simulink model "Electromech_sys_deformation"  (R2025b)
settings: Solver=VariableStepAuto  StartTime=0.0  StopTime=10.0  RelTol=1e-3
values from neighbouring files (symbols this model uses):
  p_0 = 0    [Init_Simulink_param_nl_Electromech.m]
  phat_0 = 1e-3    (= 0.001)    [Init_Simulink_param_nl_Electromech.m]
  q_0 = 0    [Init_Simulink_param_nl_Electromech.m]
  Q_0 = 0    [Init_Simulink_param_nl_Electromech.m]
  qhat_0 = 2e-4    (= 0.0002)    [Init_Simulink_param_nl_Electromech.m]
  Qhat_0 = 5e-8    (= 5e-08)    [Init_Simulink_param_nl_Electromech.m]
undefined symbols (not defined in the file or in its folder): params
settings Model: Creator=filippougolini  LastModifiedBy=filippougolini

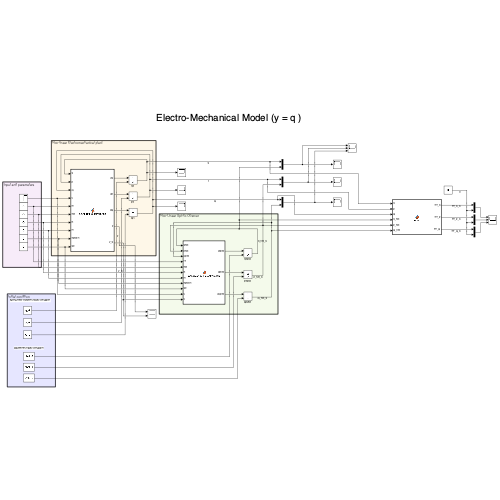
[thumbnail: Simulink's stored preview of the top-level diagram]
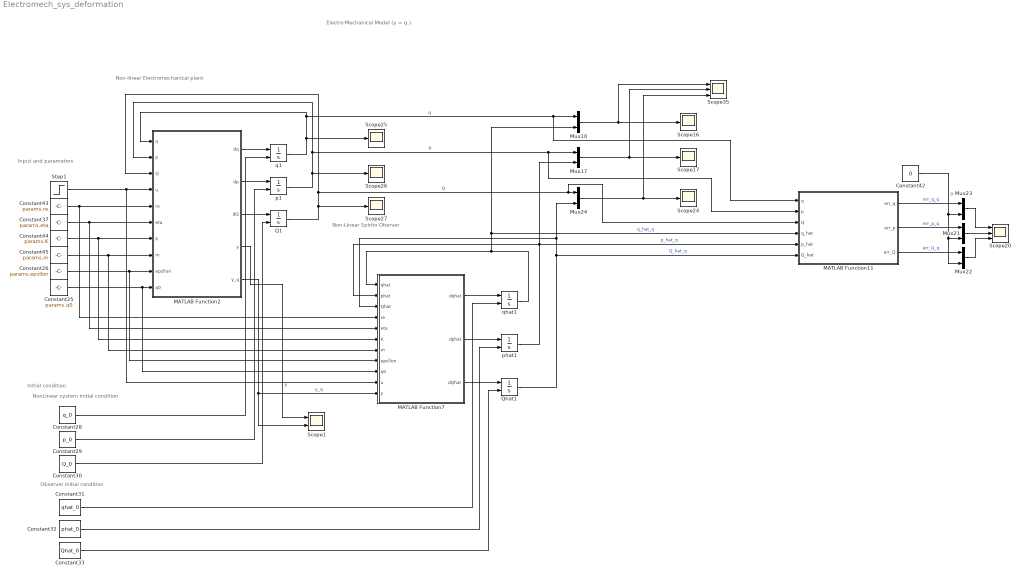
== system Electromech_sys_deformation ==
  note: Observer initial condition
  note: NonLinear system initial condition
  note: Electro-Mechanical Model (y = q )
  note: Input and parameters
  note: Non-linear Electromechanical plant
  note: Non-Linear Spirito Oberver
  note: Initial condition
  Constant25 : Constant  Value=params.q0
  Constant26 : Constant  Value=params.epsllon
  Constant28 : Constant  Value=q_0
  Constant29 : Constant  Value=p_0
  Constant30 : Constant  Value=Q_0
  Constant31 : Constant  Value=qhat_0
  Constant32 : Constant  Value=phat_0
  Constant33 : Constant  Value=Qhat_0
  Constant37 : Constant  Value=params.eta
  Constant42 : Constant  Value=0
  Constant43 : Constant  Value=params.re
  Constant44 : Constant  Value=params.K
  Constant45 : Constant  Value=params.m
  MATLAB Function11 : MATLAB Function  TreatAsAtomicUnit=on
  MATLAB Function2 : MATLAB Function  TreatAsAtomicUnit=on
  MATLAB Function7 : MATLAB Function  TreatAsAtomicUnit=on
  Mux{10,17,21..24} (6 alike) : Mux  Inputs=2
  Q1 : Integrator  InitialConditionSource=external
  Qhat1 : Integrator  InitialConditionSource=external  InitialCondition=30e-9
  Scope1 : Scope  NumInputPorts=2
      settings: ActiveDisplayYMinimum=-1  ActiveDisplayYMaximum=1
  Scope{16..17,24..27} (6 alike) : Scope
      Scope16 settings: ActiveDisplayYMinimum=-4.4929456410290065E-5  ActiveDisplayYMaximum=0.00036894675529116814  DataLoggingVariableName=ScopeData16
      Scope17 settings: ActiveDisplayYMinimum=-1  ActiveDisplayYMaximum=1  DataLoggingVariableName=ScopeData17
      Scope24 settings: ActiveDisplayYMinimum=-1  ActiveDisplayYMaximum=1  DataLoggingVariableName=ScopeData24
      Scope25 settings: ActiveDisplayYMinimum=-4.0944874698701246E-5  ActiveDisplayYMaximum=0.0003685038722883113  DataLoggingVariableName=ScopeData25
      Scope26 settings: ActiveDisplayYMinimum=-1  ActiveDisplayYMaximum=1  DataLoggingVariableName=ScopeData26
      Scope27 settings: ActiveDisplayYMinimum=-1  ActiveDisplayYMaximum=1  DataLoggingVariableName=ScopeData27
  Scope20 : Scope  NumInputPorts=3
      settings: ActiveDisplayYMinimum=-9.103686486906033E-11  ActiveDisplayYMaximum=9.2639247372251711E-11  DataLoggingVariableName=ScopeData20
  Scope35 : Scope  NumInputPorts=3
      settings: ActiveDisplayYMinimum=-4.4755980863160714E-5  ActiveDisplayYMaximum=0.00036913374297087179  DataLoggingVariableName=ScopeData35
  Step1 : Step  After=5e3  SampleTime=0
  p1 : Integrator  InitialConditionSource=external
  phat1 : Integrator  InitialConditionSource=external  InitialCondition=5e-4
  q1 : Integrator  InitialConditionSource=external
  qhat1 : Integrator  InitialConditionSource=external  InitialCondition=20e-5
  wires:
  Constant44/1 -> MATLAB Function2/7(K), MATLAB Function7/6(K)
  Constant33/1 -> Qhat1/2
  Mux17/1 -> Scope35/2, Scope17/1
  Step1/1 -> MATLAB Function7/10(u), MATLAB Function2/4(u)
  Constant37/1 -> MATLAB Function2/6(eta), MATLAB Function7/5(eta)
  MATLAB Function2/1(dq) -> q1/1
  Mux10/1 -> Scope35/1, Scope16/1
  MATLAB Function11/2(err_p) -> Mux21/1  "err_p_q"
  Constant25/1 -> MATLAB Function7/9(q0), MATLAB Function2/10(q0)
  phat1/1 -> MATLAB Function7/2(phat), MATLAB Function11/5(p_hat), Mux17/2  "p_hat_q"
  q1/1 -> Scope25/1, MATLAB Function2/1(q), Mux10/1, MATLAB Function11/1(q)  "q"
  MATLAB Function7/2(dphat) -> phat1/1
  Constant31/1 -> qhat1/2
  Constant29/1 -> p1/2
  MATLAB Function11/1(err_q) -> Mux23/1  "err_q_q"
  MATLAB Function7/1(dqhat) -> qhat1/1
  Constant45/1 -> MATLAB Function2/8(m), MATLAB Function7/7(m)
  MATLAB Function11/3(err_Q) -> Mux22/1  "err_Q_q"
  MATLAB Function7/3(dQhat) -> Qhat1/1
  Mux23/1 -> Scope20/1
  Constant32/1 -> phat1/2
  Mux21/1 -> Scope20/2
  Q1/1 -> Mux24/1, MATLAB Function11/3(Q), MATLAB Function2/3(Q), Scope27/1  "Q"
  MATLAB Function2/2(dp) -> p1/1
  Mux22/1 -> Scope20/3
  Constant30/1 -> Q1/2
  qhat1/1 -> MATLAB Function7/1(qhat), Mux10/2, MATLAB Function11/4(q_hat)  "q_hat_q"
  Constant28/1 -> q1/2
  Constant26/1 -> MATLAB Function2/9(epsllon), MATLAB Function7/8(epsllon)
  Constant43/1 -> MATLAB Function2/5(re), MATLAB Function7/4(re)
  Constant42/1 -> Mux22/2, Mux21/2, Mux23/2  "0"
  Mux24/1 -> Scope35/3, Scope24/1
  Qhat1/1 -> MATLAB Function11/6(Q_hat), Mux24/2, MATLAB Function7/3(Qhat)  "Q_hat_q"
  MATLAB Function2/3(dQ) -> Q1/1
  p1/1 -> Scope26/1, Mux17/1, MATLAB Function11/2(p), MATLAB Function2/2(p)  "p"
  MATLAB Function2/4(y) -> Scope1/1  "y"
  MATLAB Function2/5(y_q) -> Scope1/2, MATLAB Function7/11(y)  "y_q"

== matlab function Electromech_sys_deformation/MATLAB Function11 ==
  data: q input; err_q output; p input; Q input; q_hat input; p_hat input; Q_hat input; err_p output; err_Q output
function [err_q, err_p, err_Q] = error(q, p, Q, q_hat, p_hat, Q_hat)

    err_q = q - q_hat;
    err_p = p - p_hat;
    err_Q = Q - Q_hat;
end

== matlab function Electromech_sys_deformation/MATLAB Function2 ==
  data: q input; p input; Q input; u input; dq output; re input; eta input; K input; m input; epsllon input; q0 input; dp output; dQ output; y output; y_q output
function [dq, dp, dQ, y, y_q] = plant_pH_electromech(q, p, Q, u, re, eta, K, m, epsllon, q0)
% Electro-mechanical pH plant

    % Parameters: m, K, eta, eps, re, q0 in workspace

    J = [  0  1  0;
          -1  0  0;
           0  0  0 ];

    R = diag([0, eta, 1/re]);
    g = [0; 0; 1/re];

    % Hamiltonian gradient gradH(q,p,Q)
    Cq   = epsllon * (q + q0)^4;

    dHdq = K*q - 2*Q^2 / (epsllon * (q + q0)^5);
    dHdp = p / m;
    dHdQ = Q / Cq;

    gradH = [dHdq; dHdp; dHdQ];

    xdot = (J - R) * gradH + g*u;
    psi = [1/K ; 0; 2*Q/(K * (q + q0))];

    y_q = psi' * gradH; % output is the deformation
    y = q;
    
    dq = xdot(1);
    dp = xdot(2);
    dQ = xdot(3);
end

== matlab function Electromech_sys_deformation/MATLAB Function7 ==
  data: qhat input; phat input; Qhat input; re input; eta input; K input; m input; epsllon input; q0 input; u input; dqhat output; y input; dphat output; dQhat output
function [dqhat, dphat, dQhat] = observer_pH_electromech(qhat, phat, Qhat, ...
    re, eta, K, m, epsllon, q0, u, y)

    % Port-Hamiltonian structure matrices
    J = [  0  1  0;
          -1  0  0;
           0  0  0 ];

    R = diag([0, eta, 1/re]);
    g = [0; 0; 1/re];

    % -------- Hamiltonian gradient at xhat = [qhat; phat; Qhat] --------
    Cqh    = epsllon * (qhat + q0)^4;

    % dH/dqhat
    dHhdqh = K*qhat - 2*Qhat^2 / (epsllon * (qhat + q0)^5);
    % dH/dphat
    dHhdph = phat / m;
    % dH/dQhat
    dHhdQh = Qhat / Cqh;

    gradHh = [dHhdqh; dHhdph; dHhdQh];
    
    % -------- Observer gain L --------
    %Lcol = L.';       % ensure it's 3x1

    psi_hat = [1/K ; 0; 2*Qhat/(K * (qhat + q0))];

    yhat = psi_hat' * gradHh;
    alpha = 100;
    Lcol = alpha * psi_hat;
 

    % -------- Observer dynamics --------
    % Note: J and R are constant
    xhatdot = (J - R) * gradHh + g*u + Lcol * (y - yhat);

    dqhat = xhatdot(1);
    dphat = xhatdot(2);
    dQhat = xhatdot(3);
end
